simulink model "sensor_piffo"  (R2019b)
settings: Solver=VariableStepAuto  StartTime=0.0  StopTime=10.0  RelTol=1e-3
values from neighbouring files (symbols this model uses):
  Ts = evalin('base', 'Ts')    [sensors.m]
undefined symbols (not defined in the file or in its folder): sensitivity_encoder, sensitivity_giroscopio, sensors
libraries: simulink x2
settings Model: Creator=AndreaCalegari  LastModifiedBy=miche

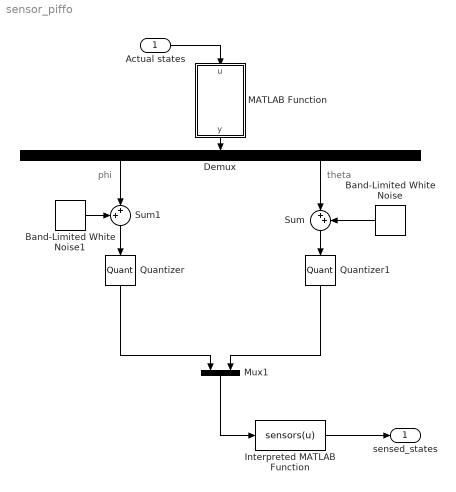
== system sensor_piffo ==
  note: phi
  note: theta
  Actual states : Inport  PortDimensions=4  SampleTime=Ts
  Band-Limited White Noise : simulink/Sources/Band-Limited White Noise  Cov=[0.00000001]  Ts=0.001  seed=[23341]
  Band-Limited White Noise1 : simulink/Sources/Band-Limited White Noise  Cov=[0.00000001]  Ts=0.001  seed=[23341]
  Demux : Demux  Outputs=2
  Interpreted MATLAB Function : MATLABFcn  MATLABFcn=sensors(u)
  MATLAB Function : MATLAB Function  TreatAsAtomicUnit=on
  Mux1 : Mux  Inputs=2
  Quantizer : Quantizer  QuantizationInterval=1/sensitivity_encoder
  Quantizer1 : Quantizer  QuantizationInterval=1/sensitivity_giroscopio
  Sum : Sum  Inputs=|++
  Sum1 : Sum  Inputs=++|
  sensed_states : Outport
  wires:
  Band-Limited White Noise/1 -> Sum/2
  MATLAB Function/1(y) -> Demux/1
  Band-Limited White Noise1/1 -> Sum1/1
  Demux/1 -> Sum1/2
  Actual states/1 -> MATLAB Function/1(u)
  Demux/2 -> Sum/1
  Sum/1 -> Quantizer1/1
  Sum1/1 -> Quantizer/1
  Quantizer1/1 -> Mux1/2
  Quantizer/1 -> Mux1/1
  Mux1/1 -> Interpreted MATLAB Function/1
  Interpreted MATLAB Function/1 -> sensed_states/1

== matlab function sensor_piffo/MATLAB Function ==
  data: u input; y output
function y = fcn(u)

y = [u(1),u(3)];
